simulink model "Problem_3"  (R2020a)
settings: Solver=VariableStepAuto  StartTime=0.0  StopTime=10.0  RelTol=1e-3
settings Model: Creator=Admin  LastModifiedBy=Admin

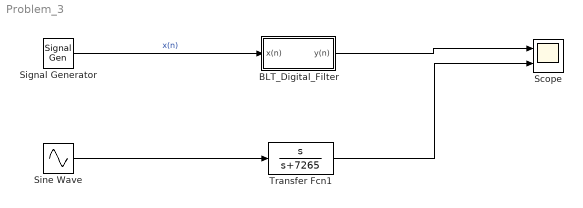
== system Problem_3 ==
  BLT_Digital_Filter : Subsystem
  Scope : Scope  NumInputPorts=2
  Signal Generator : SignalGenerator  Units=rad/sec
  Sine Wave : Sin  Frequency=3455.75  SampleTime=0
  Transfer Fcn1 : TransferFcn  Numerator=[1 0]  Denominator=[1 7265]
  wires:
  Signal Generator/1 -> BLT_Digital_Filter/1(x(n))  "x(n)"
  BLT_Digital_Filter/1(y(n)) -> Scope/1
  Transfer Fcn1/1 -> Scope/2
  Sine Wave/1 -> Transfer Fcn1/1

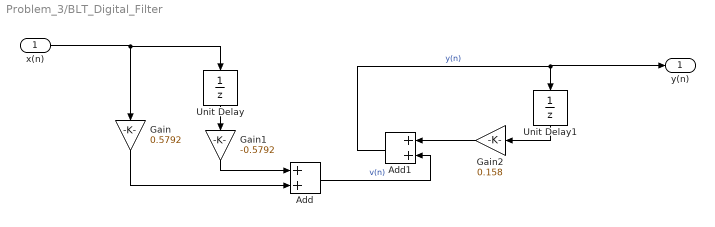
== system Problem_3/BLT_Digital_Filter ==
  x(n) : Inport
  Add : Sum
  Add1 : Sum
  Gain : Gain  Gain=0.5792
  Gain1 : Gain  Gain=-0.5792
  Gain2 : Gain  Gain=0.158
  Unit Delay : UnitDelay  SampleTime=-1  HasFrameUpgradeWarning=on
  Unit Delay1 : UnitDelay  SampleTime=-1  HasFrameUpgradeWarning=on
  y(n) : Outport
  wires:
  x(n)/1 -> Gain/1, Unit Delay/1
  Gain2/1 -> Add1/1
  Gain/1 -> Add/2
  Gain1/1 -> Add/1
  Unit Delay1/1 -> Gain2/1
  Add/1 -> Add1/2  "v(n)"
  Unit Delay/1 -> Gain1/1
  Add1/1 -> y(n)/1, Unit Delay1/1  "y(n)"
